simulink model "test_goto_from"  (R2013a)
settings: Solver=ode15s  StartTime=0.0  StopTime=0.5  MaxStep=0.001  RelTol=1e-3
libraries: fl_lib x5, nesl_utility x3
settings Model: Creator=Administrator  LastModifiedBy=Administrator
settings DebuggingCC: SolverPrmCheckMsg=none

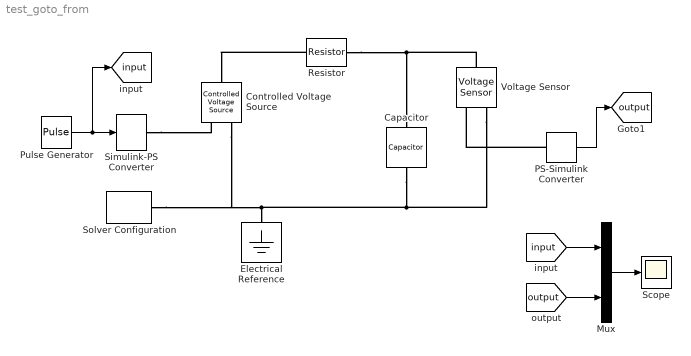
== system test_goto_from ==
  Capacitor : fl_lib/Electrical/Electrical Elements/Capacitor  c=5e-6 F  v0=0 V  r=1e-6 Ohm  g=0 1/Ohm  i_Log=off  v_Log=off  vc_Log=off  LocalVarNames=|i|v|vc  LocalVarDescs=|i|v|Internal variable for voltage across capacitor term  LocalVarLogging=[0 0 0]
  Controlled Voltage Source : fl_lib/Electrical/Electrical Sources/Controlled Voltage Source  i_Log=off  v_Log=off  LocalVarNames=|i|v  LocalVarDescs=|i|v  LocalVarLogging=[0 0]
  Electrical Reference : fl_lib/Electrical/Electrical Elements/Electrical Reference  i_Log=off  LocalVarNames=|i  LocalVarDescs=|i  LocalVarLogging=0
  Mux : Mux  Inputs=2
  PS-Simulink Converter : nesl_utility/PS-Simulink Converter  PhysicalDomain=network_engine_domain  SubClassName=ps_output  LeftPortType=input  RightPortType=output  PseudoPeriodic=off  Frequencies=[]  Unit=1  AffineConversion=off
  Pulse Generator : DiscretePulseGenerator  PulseType=Time based  Period=0.1  PulseWidth=50
  Resistor : fl_lib/Electrical/Electrical Elements/Resistor  R=1000 Ohm  i_Log=off  v_Log=off  LocalVarNames=|i|v  LocalVarDescs=|i|v  LocalVarLogging=[0 0]
  Scope : Scope
  Simulink-PS Converter : nesl_utility/Simulink-PS Converter  PhysicalDomain=network_engine_domain  SubClassName=ps_input  LeftPortType=input  RightPortType=output  PseudoPeriodic=off  Frequencies=[]  NoiseDistribution=none  NoiseParameters=[]  Unit=1  AffineConversion=off  InputFiltering=off  SimscapeFilterOrder=1  InputFilterTimeConstant=0.001  UdotUserProvided=1
  Solver Configuration : nesl_utility/Solver Configuration  PhysicalDomain=network_engine_domain  SubClassName=solver  LeftPortType=input  RightPortType=generic  Accelerate=off  Tones=[]  Harmonics=[]  SimulateNoise=off  Profile=off  UseLocalSampling=off  EnableSwitchedLinearOptims=on  FrequencyDomain=off  UseCCode=off  UseNewInitialization=off  DoDC=off  ResidualTolerance=1e-09  UseLocalSolver=off  LocalSolverChoice=NE_BACKWARD_EULER_ADVANCER  LocalSolverSampleTime=0.001  DoFixedCost=off  MaxNonlinIter=3  MaxModeIter=2  LinearAlgebra=Sparse  DelaysMemoryBudget=1024
  Voltage Sensor : fl_lib/Electrical/Electrical Sensors/Voltage Sensor  i1_Log=off  v1_Log=off  LocalVarNames=|i1|v1  LocalVarDescs=|i1|v1  LocalVarLogging=[0 0]
  tag scope: input=global, output=global
  wires:
  Pulse Generator/1 -> [input], Simulink-PS Converter/1
  Mux/1 -> Scope/1
  PS-Simulink Converter/1 -> [output]
  [input] -> Mux/1
  [output] -> Mux/2
  connections:
  Resistor/RConn1 -- Voltage Sensor/LConn1 -- Capacitor/LConn1
  Capacitor/RConn1 -- Voltage Sensor/RConn2 -- Solver Configuration/RConn1 -- Controlled Voltage Source/RConn2 -- Electrical Reference/LConn1
  Simulink-PS Converter/RConn1 -- Controlled Voltage Source/RConn1
  Resistor/LConn1 -- Controlled Voltage Source/LConn1
  PS-Simulink Converter/LConn1 -- Voltage Sensor/RConn1
